simulink model "Car24withDspace"  (R2024a)
settings: Solver=FixedStepAuto  StartTime=0.0  StopTime=Inf  FixedStep=0.001  RelTol=1e-3
PostLoadFcn:
  | if any(exist('dsrtsu_mdlpostloadfcn', 'file') ~= 0), dsrtsu_mdlpostloadfcn('Execute', bdroot); end
InitFcn:
  | , if any(exist('dsmpb_private', 'file') ~= 0), dsmpb_private('dsmpb_mdlclblib', 'Init', bdroot); end,
model workspace (MAT data in the model file):
  indicator = -1
libraries: dsmpblib x8
(part 1 of 2)
PreSaveFcn:
  | , if any(exist('dsmpb_private', 'file') ~= 0), dsmpb_private('dsmpb_mdlclblib', 'PreSave', bdroot); end,
CloseFcn:
  | , if any(exist('dsmpb_private', 'file') ~= 0), dsmpb_private('dsmpb_mdlclblib', 'Close', bdroot); end,
settings Model: DSMPB_ID_DATA={'798',struct('BlockId','ba278ee5-6691-4485-94d8-efd942a21a20','SignalIds',{{'fcd8faac-c2ce-41ea-aead-0dfdf2c47ef0'}}),'799',struct('BlockId','a8e41c90-77fc-4f06-b46f-94a13d6c991a','SignalIds',{{'22f08aa9-6fcd-41a1-b62d-e962f18854da'}}),'800',struct('BlockId','31fcda0f-fd6e-4941-ae8a-2ba19cb6e7f7','SignalIds',{{'35c98d34-17e7-4115-963b-beec5af4cec8'}}),'801',struct('BlockId','201071ae-2b6e-446e-b4ec-6a6734ee09dc','SignalIds',{{'1d100d76-8f1b-4c24-9a3c-279a1ced5831'}}),'802',struct('BlockId','a6d9fb5c-79d9-4b84-be40-f4d025ad3cea','SignalIds',{{'1cd988e0-b042-4718-91dc-4e913c3a45d9'}}),'803',struct('BlockId','53d4ca67-4f96-4e4a-b985-d2b7837ee7a0','SignalIds',{{'230ce85a-856b-4b55-a826-97e40144e857'}}),'804',struct('BlockId','a190365b-236b-46d3-8d77-caf955faebcf','SignalIds',{{'146f610b-4436-47f4-bba7-306650b5bba2'}}),'805',struct('BlockId','8fdb49cd-8d95-41ce-94e1-bab524caa5ea','SignalIds',{{'c30a0cdc-fc87-413d-a2e7-a08f688cb26a'}})}  Creator=thipp  LastModifiedBy=thipp
settings SolverCC: AutoInsertRateTranBlk=on
settings OptimizationCC: BlockReduction=off  ConditionallyExecuteInputs=off  OptimizeBlockIOStorage=off  BufferReuse=off  EnhancedBackFolding=on  PassReuseOutputArgsThreshold=0  MaxStackSize=64  OptimizeBlockOrder=speed  DifferentSizesBufferReuse=on
settings DebuggingCC: TasksWithSamePriorityMsg=none  ParameterTunabilityLossMsg=error
settings HardwareCC: ProdBitPerLong=64  ProdLargestAtomicInteger=Integer  ProdWordSize=32  ProdLongLongMode=on  ProdHWDeviceType=Custom Processor->Custom  UseEmbeddedCoderFeatures=off  UseSimulinkCoderFeatures=off
settings ModelReferenceCC: EnableParallelModelReferenceBuilds=on
settings SFSimCC: MATLABDynamicMemAlloc=off
settings RTWCC: Description=dSPACE Target DSRT - Generates SIC files for import by ConfigurationDesk and VEOS. Provides code generation for Simulink models imported in ConfigurationDesk.  SystemTargetFile=dsrt.tlc  GenCodeOnly=on  MakeCommand=make_dsrt  TemplateMakefile=dsrt_default_tmf  RTWVerbose=off  BuildConfiguration=Faster Runs
settings CodeAppCC: ForceParamTrailComments=on  OperatorAnnotations=on
settings STFCustomTargetCC: TargetLangStandard=C89/C90 (ANSI)  ParMdlRefBuildCompliant=on  GRTInterface=off  UseToolchainInfoCompliant=off  SystemTargetFile=dsrt.tlc
settings GRTTargetCC: TargetLangStandard=C89/C90 (ANSI)  CompOptLevelCompliant=off  ConcurrentExecutionCompliant=off  CombineOutputUpdateFcns=off  MatFileLogging=off  CPPClassGenCompliant=off  UseToolchainInfoCompliant=off

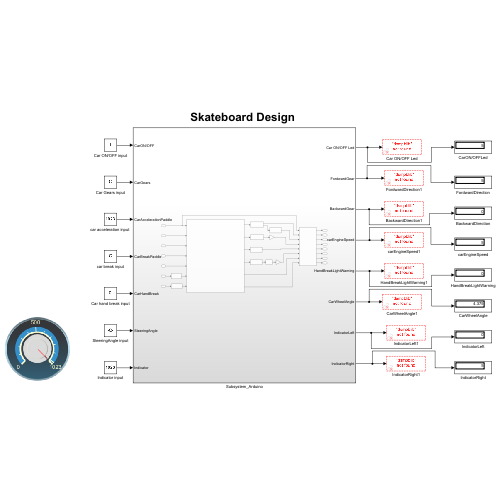
[thumbnail: Simulink's stored preview of the top-level diagram]
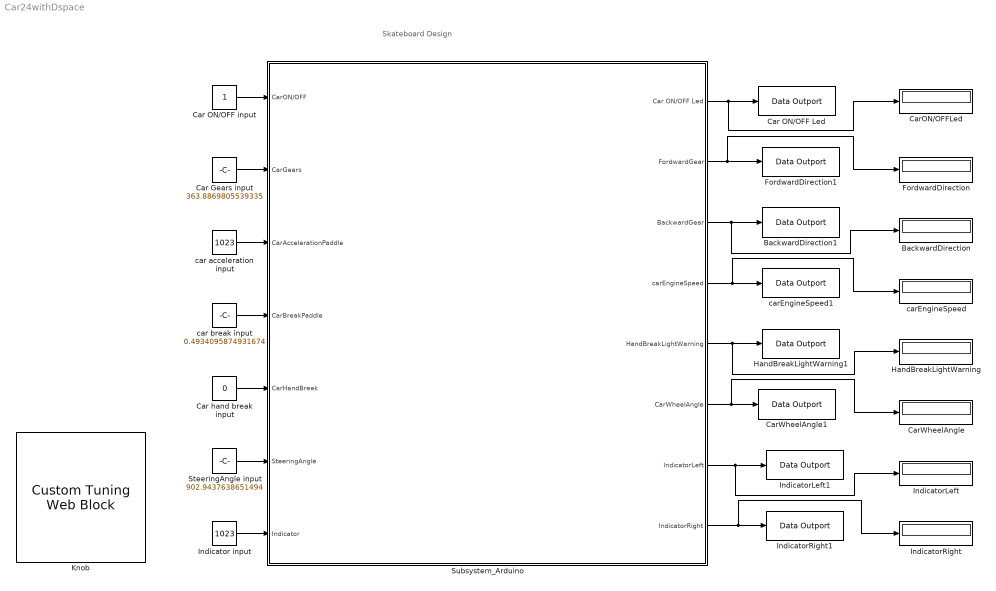
== system Car24withDspace ==
  note: Skateboard Design
  BackwardDirection : Display
  BackwardDirection1 : dsmpblib/Data Outport  Priority=-10000
      settings: SourceProductName=dSPACE Model Interface Package for Simulink (MIPS)
  Car Gears input : Constant  Value=363.8869805539335
  Car ON/OFF Led : dsmpblib/Data Outport  Priority=-10000
      settings: SourceProductName=dSPACE Model Interface Package for Simulink (MIPS)
  Car ON/OFF input : Constant
  Car hand break input : Constant  Value=0
  CarON/OFFLed : Display
  CarWheelAngle : Display
  CarWheelAngle1 : dsmpblib/Data Outport  Priority=-10000
      settings: SourceProductName=dSPACE Model Interface Package for Simulink (MIPS)
  FordwardDirection : Display
  FordwardDirection1 : dsmpblib/Data Outport  Priority=-10000
      settings: SourceProductName=dSPACE Model Interface Package for Simulink (MIPS)
  HandBreakLightWarning : Display
  HandBreakLightWarning1 : dsmpblib/Data Outport  Priority=-10000
      settings: SourceProductName=dSPACE Model Interface Package for Simulink (MIPS)
  Indicator input : Constant  Value=1023
  IndicatorLeft : Display
  IndicatorLeft1 : dsmpblib/Data Outport  Priority=-10000
      settings: SourceProductName=dSPACE Model Interface Package for Simulink (MIPS)
  IndicatorRight : Display
  IndicatorRight1 : dsmpblib/Data Outport  Priority=-10000
      settings: SourceProductName=dSPACE Model Interface Package for Simulink (MIPS)
  Knob : CustomTuningWebBlock  LabelPosition=Hide  ShowInitialText=on  Configuration="{\"components\":[{\"name\":\"CircularScaleComponent\",\"settings\":{\"bounds\":{\"max\":1023,\"min\":0,\"tickInterval\":\"auto\"},\"direction\":\"cw\",\"flipLimits\":0,\"innerRadius\":0.6636618227670849,\"internalTickHeightScaleFactor\":1,\"labelColor\":[255,255,200],\"labelFont\":{\"font\":\"Arial\",\"fontSize\":12},\"labelRadius\":0.79,\"labelTransparency\":1,\"minorTickHeightScaleFactor\":0.2,\"needleImage\":{\"size\":[150,150],\"src\":\"data:image\\/svg+xml;base64,PD94bWwgdmVyc2lvbj0iMS4wIiBlbmNvZGluZz0idXRmLTgiPz4NCjwhLS0gR2VuZXJhdG9yOiBBZG9iZSBJbGx1c3RyYXRvciAyNS4yLjMsIFNWRyBFeHBvcnQgUGx1Zy1JbiAuIFNWRyBWZXJzaW9uOiA2LjAwIEJ1aWxkIDApICAtLT4NCjxzdmcgdmVyc2lvbj0iMS4xIiBpZD0iTGF5ZXJfMSIgeG1sbnM9Imh0dHA6Ly93d3cudzMub3JnLzIwMDAvc3ZnIiB4bWxuczp4bGluaz0iaHR0cDovL3d3dy53My5vcmcvMTk5OS94bGluayIgeD0iMHB4IiB5PSIwcHgiDQoJIHZpZXdCb3g9IjAgMCAxNTIgMTUyIiBzdHlsZT0iZW5hYmxl ...(+37472 chars)\"},\"needleOffset\":[0,0],\"needleOrientation\":-45,\"needleRotation\":90,\"needleSize\":{\"height\":0.44,\"width\":0.44},\"outerRadius\":0.5053386200069245,\"position\":[0,0,1,1],\"referencePoint\":\"auto\",\"scaleAngle\":270,\"scaleAngleOffset\":135,\"scaleColors\":[],\"scaleColorsSize\":0.2,\"scaleDirection\":\"CW\",\"scalePosition\":[0,0,1,1],\"showLabels\":1,\"showMinorTicks\":1,\"showSpanLine\":true,\"showTicks\":1,\"tickColor\":[252,252,197],\"tickTransparency\":1,\"valueBarColor\":[0,114,189],\"valueBarPosition\":[0,0,1,1],\"valueBarSize\":0.2,\"valueBarTransparency\":1}},{\"name\":\"BackgroundImageComponent\",\"settings\":{\"image\":{\"size\":[385,373],\"src\":\"data:image\\/svg+xml;base64,PD94bWwgdmVyc2lvbj0iMS4wIiBlbmNvZGluZz0idXRmLTgiPz4NCjwhLS0gR2VuZXJhdG9yOiBBZG9iZSBJbGx1c3RyYXRvciAyNS4wLjAsIFNWRyBFeHBvcnQgUGx1Zy1JbiAuIFNWRyBWZXJzaW9uOiA2LjAwIEJ1aWxkIDApICAtLT4NCjxzdmcgdmVyc2lvbj0iMS4xIg0KCSBpZD0iTGF5ZXJfMl8xXyIgeG1sbnM6Y2M9Imh0dHA6Ly9jcmVhdGl2ZWNvbW1vbnMub3JnL25zIyIgeG1sbnM6ZGM9Imh0dHA6Ly9wdXJsLm9yZy9kYy9lbGVtZW50cy8xLjEvIiB4bWxuczppbmtzY2FwZT0iaHR0cDovL3d3dy5pbmtzY2FwZS5vcmcv ...(+4184 chars)\",\"srcOrientation\":\"horizontal\"},\"position\":[0,0,1,1],\"scaleMode\":\"0\"}},{\"name\":\"ForegroundImageComponent\",\"settings\":{\"image\":{\"size\":[0,0],\"src\":\"default\",\"srcOrientation\":[]},\"isForeground\":1,\"position\":[0,0,1,1],\"scaleMode\":\"0\"}}],\"settings\":{\"BindingType\":\"param\",\"aspectRatio\":1,\"backgroundColor\":[0,0,0,\"1\"],\"backgroundOffset\":1,\"backgroundOpacity\":1,\"direction\":\"cw\",\"fixedAspectRatio\":\"on\",\"flipLimits\":0,\"foregroundColor\":[252,252,196],\"orientation\":\"horizontal\",\"showBackgroundColor\":false,\"value\":0,\"version\":\"R2023a\"},\"type\":\"CircularGauge\"}"
  SteeringAngle input : Constant  Value=902.9437638651494
  Subsystem_Arduino : Subsystem
  "car acceleration input " : Constant  Value=1023
  car break input : Constant  Value=0.4934095874931674
  carEngineSpeed : Display
  carEngineSpeed1 : dsmpblib/Data Outport  Priority=-10000
      settings: SourceProductName=dSPACE Model Interface Package for Simulink (MIPS)
  wires:
  Subsystem_Arduino/3(BackwardGear) -> BackwardDirection1/1, BackwardDirection/1
  Subsystem_Arduino/4(carEngineSpeed) -> carEngineSpeed1/1, carEngineSpeed/1
  Subsystem_Arduino/5(HandBreakLightWarning) -> HandBreakLightWarning1/1, HandBreakLightWarning/1
  Subsystem_Arduino/6(CarWheelAngle) -> CarWheelAngle1/1, CarWheelAngle/1
  Subsystem_Arduino/7(IndicatorLeft) -> IndicatorLeft1/1, IndicatorLeft/1
  Subsystem_Arduino/8(IndicatorRight) -> IndicatorRight1/1, IndicatorRight/1
  Subsystem_Arduino/1(Car ON/OFF Led) -> Car ON/OFF Led/1, CarON/OFFLed/1
  Car Gears input/1 -> Subsystem_Arduino/2(CarGears)
  car break input/1 -> Subsystem_Arduino/4(CarBreakPaddle)
  SteeringAngle input/1 -> Subsystem_Arduino/6(SteeringAngle)
  Car ON/OFF input/1 -> Subsystem_Arduino/1(CarON/OFF)
  Car hand break input/1 -> Subsystem_Arduino/5("CarHandBreak ")
  Indicator input/1 -> Subsystem_Arduino/7(Indicator)
  "car acceleration input "/1 -> Subsystem_Arduino/3(CarAccelerationPaddle)
  Subsystem_Arduino/2(FordwardGear) -> FordwardDirection1/1, FordwardDirection/1
